simulink model "schemadubled"  (R2020b)
settings: Solver=VariableStepAuto  StartTime=0.0  StopTime=1  RelTol=1e-3
values from neighbouring files (symbols this model uses):
  Kc = 0.58    [Initialisation_variable.m]
  Kv = 0.58    [Initialisation_variable.m]
  LJ = L*J    (= 5e-06)    [Initialisation_variable.m]
  Ly = L*y    (= 5e-06)    [Initialisation_variable.m]
  RJ = R*J    (= 0.00444)    [Initialisation_variable.m]
  Ry = R*y    (= 0.00444)    [Initialisation_variable.m]
settings Model: Creator=Etudiants  LastModifiedBy=Etudiants

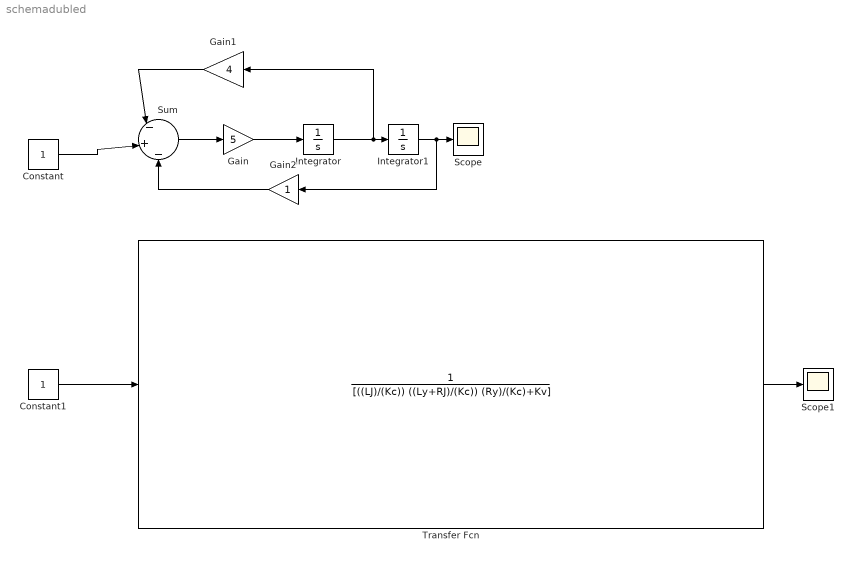
== system schemadubled ==
  Constant : Constant
  Constant1 : Constant
  Gain : Gain  Gain=5
  Gain1 : Gain  Gain=4
  Gain2 : Gain
  Integrator : Integrator
  Integrator1 : Integrator
  Scope : Scope
  Scope1 : Scope
  Sum : Sum  Inputs=|-|+|-
  Transfer Fcn : TransferFcn  Denominator=[((LJ)/(Kc)) ((Ly+RJ)/(Kc)) (Ry)/(Kc)+Kv]
  wires:
  Sum/1 -> Gain/1
  Gain/1 -> Integrator/1
  Integrator/1 -> Integrator1/1, Gain1/1
  Integrator1/1 -> Scope/1, Gain2/1
  Gain1/1 -> Sum/1
  Gain2/1 -> Sum/3
  Constant/1 -> Sum/2
  Transfer Fcn/1 -> Scope1/1
  Constant1/1 -> Transfer Fcn/1
